simulink model "test"  (R2020a)
settings: Solver=VariableStepAuto  StartTime=0.0  StopTime=stop_time  RelTol=1e-3
InitFcn:
  | [input_wav_signal, Fs_in] = audioread('Acoustic.wav');
  | 
  | signal = resample(input_wav_signal, 48000, 11025);
  | 
  | Fs = 48000;
  | Ts = 1/Fs;
  | 
  | Fs_system = Fs*2;
  | Ts_system = 1/Fs_system;
  | 
  | timevals = [0:length(signal)-1]*Ts;
  | input_signal =timeseries(signal,timevals);
  | 
  | stop_time =length(signal)*Ts;
  | 
  | W_bits = 32;
  | F_bits = 28;
  | 
  | index=1:length(signal);
  | 
  | figure(1);
  | plot(signal)
StopFcn:
  | yout = output_signal.Data(:);
  | 
  | figure(2);
  | plot(yout)
  | soundsc(yout, Fs_system);
  | audiowrite("simulink_tremolo.wav",yout, Fs_system);
libraries: dspsrcs4 x1
settings Model: Creator=Owner  LastModifiedBy=Owner
settings DataIOCC: ReturnWorkspaceOutputs=off

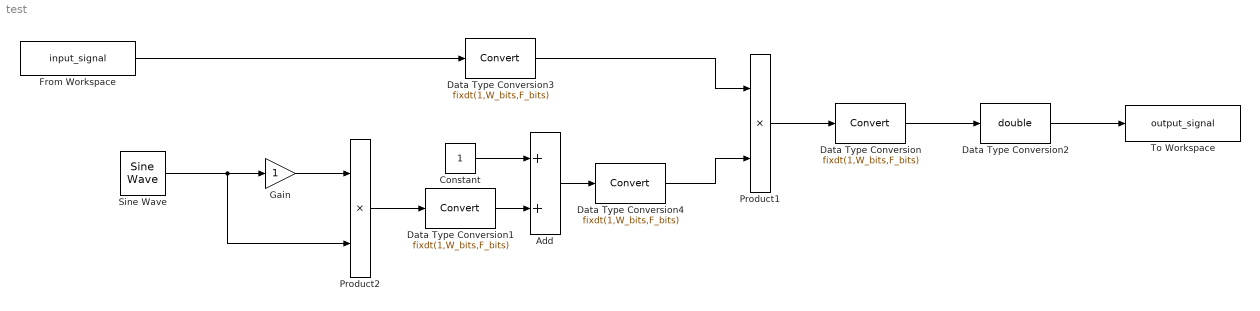
== system test ==
  Add : Sum  OutDataTypeStr=fixdt(1,W_bits,F_bits)
  Constant : Constant  OutDataTypeStr=fixdt(1,W_bits,F_bits)  SampleTime=Ts_system
  Data Type Conversion{,1,3..4} (4 alike) : DataTypeConversion  OutDataTypeStr=fixdt(1,W_bits,F_bits)  RndMeth=Nearest
  Data Type Conversion2 : DataTypeConversion  OutDataTypeStr=double  RndMeth=Nearest
  From Workspace : FromWorkspace  VariableName=input_signal  SampleTime=Ts_system
  Gain : Gain
  Product1 : Product
  Product2 : Product
  Sine Wave : dspsrcs4/Sine Wave  Amplitude=1  Frequency=5  Phase=0  SampleMode=Discrete  OutComplex=Real  CompMethod=Table lookup  TableSize=Speed  SampleTime=Ts_system  SamplesPerFrame=1  ResetState=Restart at time zero  OutputFrames=off  dataType=Fixed-point  wordLen=32  udDataType=sfix(16)  fracBitsMode=User-defined  numFracBits=28  OutDataTypeStr=fixdt(1,32,28)  LastOutDataTypeStr=fixdt(1,32,28)
  To Workspace : ToWorkspace  VariableName=output_signal  SaveFormat=Timeseries  SampleTime=-1
  wires:
  Data Type Conversion1/1 -> Add/2
  Data Type Conversion/1 -> Data Type Conversion2/1
  Product1/1 -> Data Type Conversion/1
  Product2/1 -> Data Type Conversion1/1
  Constant/1 -> Add/1
  Data Type Conversion2/1 -> To Workspace/1
  Add/1 -> Data Type Conversion4/1
  Data Type Conversion4/1 -> Product1/2
  Data Type Conversion3/1 -> Product1/1
  From Workspace/1 -> Data Type Conversion3/1
  Gain/1 -> Product2/1
  Sine Wave/1 -> Product2/2, Gain/1
